simulink subsystem "Battery"  (R2025a)
settings: Solver=VariableStepAuto  StartTime=0.0  StopTime=10  RelTol=1e-3
model mask{minSOC=0, maxSOC=0, energyRating=0, capacityRating=0, nominalVoltage=0, frequency=0, windingRatio=0}
  mask prompts: minSOC "Minimum Operating SOC"; maxSOC "Maximum Operating SOC"; energyRating "Energy rating (kWh)"; capacityRating "Capacity Rating (Ah)"; nominalVoltage "Nominal Voltage (V)"; frequency "Frequency (Hz)"; windingRatio "Transformer Ratio"
libraries: fl_lib x13, ee_lib x6, nesl_utility x5, simulink x2, batteryecm_lib x1, eeGeneralControl x1
settings Model: DefaultTestHarness=Battery_Harness  Creator=skota  LastModifiedBy=skota

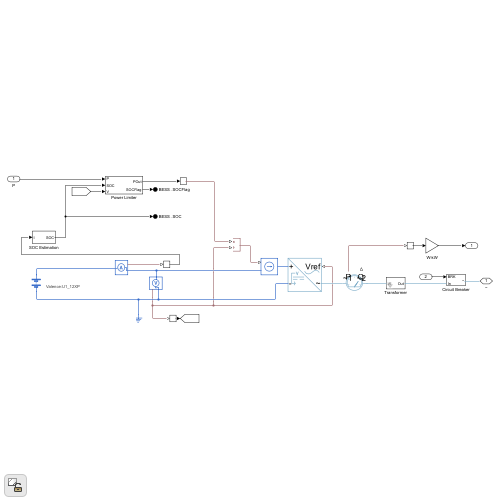
[thumbnail: Simulink's stored preview of the top-level diagram]
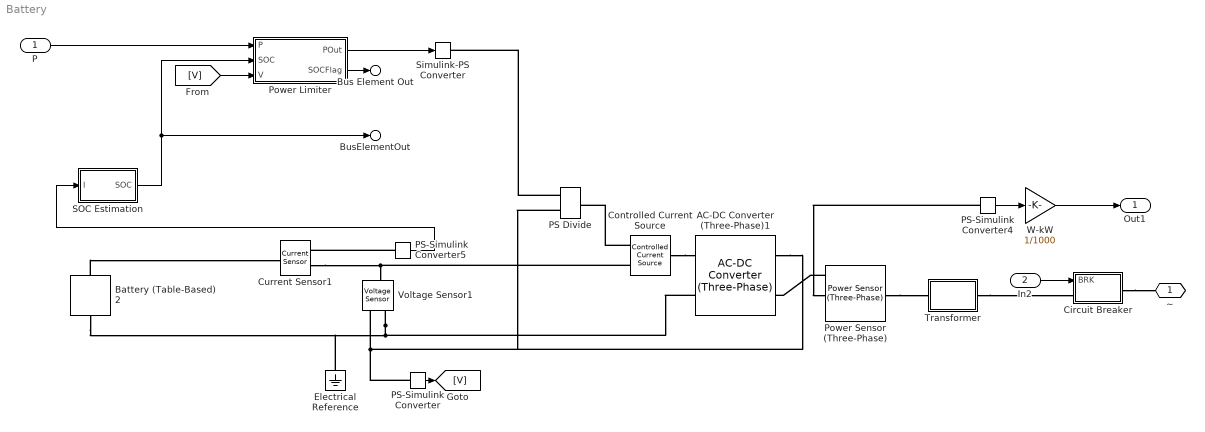
== system Battery ==
  P : Inport
  In2 : Inport  Port=2
  AC-DC Converter (Three-Phase)1 : ee_lib/Semiconductors & Converters/Converters/AC-DC Converter (Three-Phase)  port_option=ee.enum.threePhasePort.composite  droop=0.001 V/A  Vdc_dynamics=ee.enum.converters.dynamics.no  tauVdc=0.02 s  Vdc_ini=100 V  FRated=frequency Hz  Vline_rms_min=0.1 V  tauVac=1e-3 s  Vline_rms_ini=10000 V  Vang_ini=0 deg  power_dynamics=ee.enum.converters.powerDynamics.no  tauP=0.01 s  P_ini=1e3 W  gmin=1e-4 S
      settings: InternalSimscapePortConfiguration="{\"Bottom\":[],\"Left\":[{\"id\":\"Vref\",\"label\":\"Vref\",\"type\":\"input\"},{\"id\":\"N\",\"label\":\"~\",\"type\":\"foundation.electrical.three_phase\"}],\"Right\":[{\"id\":\"p\",\"label\":\"+\",\"type\":\"foundation.electrical.electrical\"},{\"id\":\"n\",\"label\":\"-\",\"type\":\"foundation.electrical.electrical\"}],\"Top\":[]}"
  Battery (Table-Based)2 : batteryecm_lib/Battery (Table-Based)  Tag={'toolbox/physmod/battery/shared_library/m/batteryecm_lib_parts';'Battery__Table_Based_/Valence/U1_12XP.xml'}  SOC_vec=[0 0.01 0.02 0.03 0.04 0.05 0.06 0.07 0.08 0.09 0.1 0.11 0.12 0.13 0.14 0.15 0.16 0.17 0.18 0.19 0.2 0.21 0.22 0.23 0.24 0.25 0.26 0.27 0.28 0.29 0.3 0.31 0.32 0.33 0.34 0.35 0.36 0.37 0.38 0.39 0.4 0.41 0.42 0.43 0.44 0.45 0.46 0.47 0.48 0.49 0.5 0.51 0.52 0.53 0.54 0.55 0.56 0.57 0.58 0.59 0.6 0.61 0.62 0.63 0.64 0.65 0.66 0.67 0.68 0.69 0.7 0.71 0.72 0.73 0.74 0.75 0.76 0.77 0.78 0.79 0.8 0.81 0.82 0.83 0.84 0.85 0.86 0.87 0.88 0.89 0.9 0.91 0.92 0.93 0.94 0.95 0.96 0.97 0.98 0.99 1]  T_dependence=simscape.enum.tablebattery.temperature_dependence.no  prm_dir=simscape.enum.tablebattery.prm_dir.noCurrentDirectionality  T_vec=[-10 0 10 20 23 30 40] degC  V0_mat=[12.00518 12.00518 12.00518 12.00518 12.00518 12.00518 12.00518;12.046 12.046 12.046 12.046 12.046 12.046 12.046;12.08682 12.08682 12.08682 12.08682 12.08682 12.08682 12.08682;12.12763 12.12763 12.12763 12.12763 12.12763 12.12763 12.12763;12.16845 12.16845 12.16845 12.16845 12.16845 12.16845 12.16845;12.20927 12.20927 12.20927 12.20927 12.20927 12.20927 12.20927;12.25009 12.25009 12.25009 12.25009 12.25009 12.25009 12.25009;12.29091 12.29091 12.29091 12.29091 12.29091 12.29091 12.29091;12.33173 12.33173 12.33173 12.33173 12.33173 12.33173 12.33173;12.37255 12.37255 12.37255 12.37255 12.37255 12.37255 12.37255;12.41337 12.41337 12.41337 12.41337 12.41337 12.41337 12.41337;12.45419 12.45419 12.45419 12.45419 12.45419 12.45419 12.45419;12.49501 12.49501 12.49501 12.49501 12.49501 12.49501 12.49501;12.53583 12.53583 12.53583 12.53583 12.53583 12.53583 12.53583;12.56952 12.56952 12.56952 12.56952 12.56952 12.56952 12.56952;12.60149 12.60149 12.60149 12.60149 12.60149 12.60149 12.60149;12.63628 12.63628 12.63628 12.63628 12.63628 12.63628 12.63628;12.66676 12.66676 12.66676 12.66676 12.66676 12.66676 12.66676;12.6925 12.6925 12.6925 12.6925 12.6925 12.6925 12.6925;12.71984 12.71984 12.71984 12.71984 12.71984 12.71984 12.71984;12.74668 12.74668 12.74668 12.74668 12.74668 12.74668 12.74668;12.7709 12.7709 12.7709 12.7709 12.7709 12.7709 12.7709;12.79145 12.79145 12.79145 12.79145 12.79145 12.79145 12.79145;12.81167 12.81167 12.81167 12.81167 12.81167 12.81167 12.81167;12.82987 12.82987 12.82987 12.82987 12.82987 12.82987 12.82987;12.84554 12.84554 12.84554 12.84554 12.84554 12.84554 12.84554;12.85927 12.85927 12.85927 12.85927 12.85927 12.85927 12.85927;12.87336 12.87336 12.87336 12.87336 12.87336 12.87336 12.87336;12.8878 12.8878 12.8878 12.8878 12.8878 12.8878 12.8878;12.90226 12.90226 12.90226 12.90226 12.90226 12.90226 12.90226;12.91618 12.91618 12.91618 12.91618 12.91618 12.91618 12.91618;12.92892 12.92892 12.92892 12.92892 12.92892 12.92892 12.92892;12.9409 12.9409 12.9409 12.9409 12.9409 12.9409 12.9409;12.95179 12.95179 12.95179 12.95179 12.95179 12.95179 12.95179;12.96212 12.96212 12.96212 12.96212 12.96212 12.96212 12.96212;12.9718 12.9718 12.9718 12.9718 12.9718 12.9718 12.9718;12.98121 12.98121 12.98121 12.98121 12.98121 12.98121 12.98121;12.9894 12.9894 12.9894 12.9894 12.9894 12.9894 12.9894;12.99628 12.99628 12.99628 12.99628 12.99628 12.99628 12.99628;13.00194 13.00194 13.00194 13.00194 13.00194 13.00194 13.00194;13.00687 13.00687 13.00687 13.00687 13.00687 13.00687 13.00687;13.01127 13.01127 13.01127 13.01127 13.01127 13.01127 13.01127;13.01612 13.01612 13.01612 13.01612 13.01612 13.01612 13.01612;13.0201 13.0201 13.0201 13.0201 13.0201 13.0201 13.0201;13.0231 13.0231 13.0231 13.0231 13.0231 13.0231 13.0231;13.0261 13.0261 13.0261 13.0261 13.0261 13.0261 13.0261;13.02911 13.02911 13.02911 13.02911 13.02911 13.02911 13.02911;13.03211 13.03211 13.03211 13.03211 13.03211 13.03211 13.03211;13.03451 13.03451 13.03451 13.03451 13.03451 13.03451 13.03451;13.03664 13.03664 13.03664 13.03664 13.03664 13.03664 13.03664;13.03933 13.03933 13.03933 13.03933 13.03933 13.03933 13.03933;13.04232 13.04232 13.04232 13.04232 13.04232 13.04232 13.04232;13.04573 13.04573 13.04573 13.04573 13.04573 13.04573 13.04573;13.04919 13.04919 13.04919 13.04919 13.04919 13.04919 13.04919;13.05277 13.05277 13.05277 13.05277 13.05277 13.05277 13.05277;13.05642 13.05642 13.05642 13.05642 13.05642 13.05642 13.05642;13.06013 13.06013 13.06013 13.06013 13.06013 13.06013 13.06013;13.06395 13.06395 13.06395 13.06395 13.06395 13.06395 13.06395;13.06828 13.06828 13.06828 13.06828 13.06828 13.06828 13.06828;13.07261 13.07261 13.07261 13.07261 13.07261 13.07261 13.07261;13.07686 13.07686 13.07686 13.07686 13.07686 13.07686 13.07686;13.08121 13.08121 13.08121 13.08121 13.08121 13.08121 13.08121;13.08594 13.08594 13.08594 13.08594 13.08594 13.08594 13.08594;13.09142 13.09142 13.09142 13.09142 13.09142 13.09142 13.09142;13.09708 13.09708 13.09708 13.09708 ...(+2253 chars)] V  V0_vec=[12.00518 12.046 12.08682 12.12763 12.16845 12.20927 12.25009 12.29091 12.33173 12.37255 12.41337 12.45419 12.49501 12.53583 12.56952 12.60149 12.63628 12.66676 12.6925 12.71984 12.74668 12.7709 12.79145 12.81167 12.82987 12.84554 12.85927 12.87336 12.8878 12.90226 12.91618 12.92892 12.9409 12.95179 12.96212 12.9718 12.98121 12.9894 12.99628 13.00194 13.00687 13.01127 13.01612 13.0201 13.0231 13.0261 13.02911 13.03211 13.03451 13.03664 13.03933 13.04232 13.04573 13.04919 13.05277 13.05642 13.06013 13.06395 13.06828 13.07261 13.07686 13.08121 13.08594 13.09142 13.09708 13.10279 13.10857 13.11438 13.12019 13.1263 13.13263 13.13899 13.14595 13.15268 13.15967 13.16669 13.17384 13.17943 13.18402 13.18838 13.19255 13.19694 13.20123 13.20527 13.20912 13.2115 13.21389 13.21588 13.21758 13.21949 13.22126 13.224 13.227 13.23066 13.23444 13.23732 13.23875 13.23911 13.23888 13.25149 13.31471]*100 V  V_range=[9 Inf] V  R0_mat=[0.31149 0.24646 0.1305 0.14557 0.06981 0.12094 0.10043;0.31245 0.23652 0.11852 0.12502 0.0625 0.09416 0.06761;0.30299 0.22658 0.10654 0.10446 0.05518 0.071 0.05004;0.29352 0.21664 0.09456 0.08497 0.04785 0.05545 0.03565;0.28405 0.2067 0.08326 0.0695 0.04083 0.04376 0.02394;0.27458 0.19676 0.07425 0.05748 0.03437 0.03259 0.01541;0.26512 0.18683 0.06508 0.0482 0.02911 0.02462 0.00923;0.25565 0.17689 0.05699 0.04095 0.02515 0.01945 0.00517;0.24618 0.16695 0.05025 0.03428 0.02195 0.01534 0.00236;0.23671 0.15701 0.04492 0.02949 0.01956 0.0115 0.00085;0.22724 0.14707 0.04118 0.02542 0.01764 0.00986 0.00061;0.21778 0.13713 0.03744 0.02233 0.01618 0.00823 0.00064;0.20831 0.12719 0.03369 0.01978 0.01518 0.00787 0.00119;0.19884 0.11725 0.03108 0.01847 0.01436 0.00758 0.00174;0.18937 0.10701 0.0287 0.01681 0.01349 0.00698 0.00186;0.1799 0.09743 0.02624 0.01521 0.01311 0.00656 0.00189;0.17044 0.08843 0.02418 0.01493 0.01277 0.00629 0.00207;0.16097 0.08111 0.0236 0.01443 0.01245 0.00644 0.00225;0.1515 0.074 0.02279 0.01369 0.01206 0.00666 0.00245;0.14203 0.0677 0.02206 0.01303 0.01189 0.00696 0.00273;0.13257 0.06168 0.0213 0.01283 0.01179 0.00725 0.00299;0.12217 0.05582 0.02087 0.01288 0.01168 0.00749 0.00323;0.11213 0.0525 0.02085 0.01275 0.01153 0.00754 0.00344;0.10314 0.04948 0.02082 0.0126 0.01152 0.00757 0.00364;0.09444 0.04636 0.02069 0.01235 0.01151 0.0075 0.00376;0.08561 0.04418 0.02043 0.01214 0.01146 0.00748 0.0039;0.07908 0.04215 0.02007 0.01218 0.0114 0.00741 0.00395;0.073 0.04014 0.01973 0.01225 0.01137 0.00737 0.00401;0.06878 0.03834 0.01964 0.01233 0.01137 0.00734 0.00403;0.06496 0.03708 0.01958 0.01241 0.01138 0.00731 0.00405;0.06117 0.0358 0.01949 0.01246 0.0114 0.00726 0.00405;0.05837 0.03446 0.01935 0.01262 0.01143 0.00716 0.00415;0.05554 0.0331 0.01917 0.01274 0.01146 0.00743 0.00426;0.05334 0.0326 0.01893 0.01281 0.01148 0.00765 0.00437;0.05171 0.03208 0.01888 0.01285 0.01149 0.00784 0.00451;0.05005 0.03152 0.01897 0.01286 0.0115 0.00799 0.00462;0.04837 0.03123 0.01906 0.01285 0.01151 0.00813 0.00474;0.04707 0.03089 0.01908 0.01288 0.01153 0.00821 0.00481;0.04632 0.03049 0.01903 0.01286 0.01152 0.00823 0.00482;0.04552 0.03007 0.01892 0.01278 0.0115 0.00818 0.00477;0.04468 0.02982 0.01878 0.01267 0.01147 0.00814 0.00471;0.04381 0.02954 0.01861 0.01253 0.01143 0.00809 0.00463;0.04296 0.02929 0.01847 0.01241 0.01141 0.00807 0.00457;0.04221 0.02899 0.0184 0.01224 0.01138 0.008 0.00447;0.04182 0.02866 0.01828 0.01203 0.01134 0.00789 0.00432;0.04143 0.02837 0.01816 0.01182 0.0113 0.00777 0.00417;0.04103 0.02807 0.01804 0.01172 0.01126 0.00767 0.00402;0.04064 0.02778 0.01792 0.01163 0.01122 0.00757 0.00401;0.04022 0.02746 0.01777 0.0115 0.01117 0.00745 0.00397;0.03979 0.02712 0.0176 0.01136 0.01113 0.00731 0.00391;0.03964 0.02688 0.01747 0.01125 0.0111 0.0072 0.00389;0.03949 0.02672 0.01735 0.01116 0.01108 0.0071 0.00387;0.03937 0.02658 0.01725 0.01108 0.01106 0.00705 0.00387;0.03925 0.02644 0.01717 0.01101 0.01105 0.00699 0.00387;0.03914 0.02631 0.01711 0.01094 0.01104 0.00695 0.00385;0.03903 0.02618 0.01705 0.01092 0.01103 0.0069 0.00384;0.03892 0.0262 0.017 0.01089 0.01102 0.00686 0.00382;0.03882 0.02624 0.01695 0.01087 0.01101 0.00683 0.00382;0.03877 0.02629 0.01693 0.01088 0.01102 0.00683 0.00387;0.0389 0.02635 0.01691 0.01089 0.01104 0.00684 0.00391;0.03901 0.0264 0.01689 0.01089 0.01105 0.00685 0.00396;0.03914 0.02644 0.01687 0.0109 0.01107 0.00686 0.004;0.03928 0.02648 0.01687 0.01093 0.01109 0.00689 0.00407;0.03946 0.02656 0.01694 0.011 0.01113 0.00695 0.00415;0.03965 0.02665 0.01709 0.01108 0.01117 0.00703 0.00425;0.03995 0.02674 0.01724 0.01117 0.01122 0.00714 0.00434;0.04035 0.02683 0.01739 0.01126 0.01127 0.00725 0.00443;0.04075 0.02692 0.01754 0.01136 0.01131 0.00736 0.00452;0.04115 0.02711 0.0177 0.01145 0.01136 0.00747 0.00461;0.04157 0.02734 0.01787 0.01156 0.01142 0.00759 0.00472;0.04196 0.02759 0.01803 0.01168 0.01148 0.00773 0.00483;0.04232 0.02783 0.01813 0.01181 0.01153 0.00786 0.00495;0.04271 0.02811 ...(+1584 chars)] Ohm  R0_vec=[0.06981 0.0625 0.05518 0.04785 0.04083 0.03437 0.02911 0.02515 0.02195 0.01956 0.01764 0.01618 0.01518 0.01436 0.01349 0.01311 0.01277 0.01245 0.01206 0.01189 0.01179 0.01168 0.01153 0.01152 0.01151 0.01146 0.0114 0.01137 0.01137 0.01138 0.0114 0.01143 0.01146 0.01148 0.01149 0.0115 0.01151 0.01153 0.01152 0.0115 0.01147 0.01143 0.01141 0.01138 0.01134 0.0113 0.01126 0.01122 0.01117 0.01113 0.0111 0.01108 0.01106 0.01105 0.01104 0.01103 0.01102 0.01101 0.01102 0.01104 0.01105 0.01107 0.01109 0.01113 0.01117 0.01122 0.01127 0.01131 0.01136 0.01142 0.01148 0.01153 0.0116 0.01166 0.01174 0.01182 0.0119 0.01195 0.012 0.01204 0.01209 0.01214 0.01219 0.01223 0.01227 0.01226 0.01225 0.01223 0.01221 0.01217 0.01212 0.01208 0.01205 0.01201 0.01196 0.01184 0.0117 0.01136 0.01069 0.0098 0.00774] Ohm  R0_dis_mat=[.0117, .0085, .009; .011, .0085, .009; .0114, .0087, .0092; .0107, .0082, .0088; .0107, .0083, .0091; .0113, .0085, .0089; .0116, .0085, .0089] % Parameter not set Ohm  R0_dis_vec=[.0085, .0085, .0087, .0082, .0083, .0085, .0085] % Parameter not set Ohm  R0_ch_mat=[.0117, .0085, .009; .011, .0085, .009; .0114, .0087, .0092; .0107, .0082, .0088; .0107, .0083, .0091; .0113, .0085, .0089; .0116, .0085, .0089] % Parameter not set Ohm  R0_ch_vec=[.0085, .0085, .0087, .0082, .0083, .0085, .0085] % Parameter not set Ohm  AH=40.779*ceil(energyRating*1000/(nominalVoltage*capacityRating)) hr*A  prm_leak=simscape.enum.tablebattery.prm_leak.disabled  Rleak_vec=[8000, 7000, 6000] % Parameter not set Ohm  Rleak=7e3 % Parameter not set Ohm  extrapolation_option=simscape.enum.extrapolation.nearest  SOC_port=simscape.enum.tablebattery.enable.no  prm_dyn=simscape.enum.tablebattery.prm_dyn.off  R1_mat=[.0109, .0029, .0013; .0069, .0024, .0012; .0047, .0026, .0013; .0034, .0016, .001; .0033, .0023, .0014; .0033, .0018, .0011; .0028, .0017, .0011] % Parameter not set Ohm  R1_vec=[.0029, .0024, .0026, .0016, .0023, .0018, .0017] % Parameter not set Ohm  tau1_mat=[20, 36, 39; 31, 45, 39; 109, 105, 61; 36, 29, 26; 59, 77, 67; 40, 33, 29; 25, 39, 33] % Parameter not set s  tau1_vec=[36, 45, 105, 29, 77, 33, 39] % Parameter not set s  R2_mat=[.0109, .0029, .0013; .0069, .0024, .0012; .0047, .0026, .0013; .0034, .0016, .001; .0033, .0023, .0014; .0033, .0018, .0011; .0028, .0017, .0011] % Parameter not set Ohm  R2_vec=[.0029, .0024, .0026, .0016, .0023, .0018, .0017] % Parameter not set Ohm  tau2_mat=[20, 36, 39; 31, 45, 39; 109, 105, 61; 36, 29, 26; 59, 77, 67; 40, 33, 29; 25, 39, 33] % Parameter not set s  tau2_vec=[36, 45, 105, 29, 77, 33, 39] % Parameter not set s  R3_mat=[.0109, .0029, .0013; .0069, .0024, .0012; .0047, .0026, .0013; .0034, .0016, .001; .0033, .0023, .0014; .0033, .0018, .0011; .0028, .0017, .0011] % Parameter not set Ohm  R3_vec=[.0029, .0024, .0026, .0016, .0023, .0018, .0017] % Parameter not set Ohm  tau3_mat=[20, 36, 39; 31, 45, 39; 109, 105, 61; 36, 29, 26; 59, 77, 67; 40, 33, 29; 25, 39, 33] % Parameter not set s  tau3_vec=[36, 45, 105, 29, 77, 33, 39] % Parameter not set s  R4_mat=[.0109, .0029, .0013; .0069, .0024, .0012; .0047, .0026, .0013; .0034, .0016, .001; .0033, .0023, .0014; .0033, .0018, .0011; .0028, .0017, .0011] % Parameter not set Ohm  R4_vec=[.0029, .0024, .0026, .0016, .0023, .0018, .0017] % Parameter not set Ohm  tau4_mat=[20, 36, 39; 31, 45, 39; 109, 105, 61; 36, 29, 26; 59, 77, 67; 40, 33, 29; 25, 39, 33] % Parameter not set s  tau4_vec=[36, 45, 105, 29, 77, 33, 39] % Parameter not set s  R5_mat=[.0109, .0029, .0013; .0069, .0024, .0012; .0047, .0026, .0013; .0034, .0016, .001; .0033, .0023, .0014; .0033, .0018, .0011; .0028, .0017, .0011] % Parameter not set Ohm  R5_vec=[.0029, .0024, .0026, .0016, .0023, .0018, .0017] % Parameter not set Ohm  tau5_mat=[20, 36, 39; 31, 45, 39; 109, 105, 61; 36, 29, 26; 59, 77, 67; 40, 33, 29; 25, 39, 33] % Parameter not set s  tau5_vec=[36, 45, 105, 29, 77, 33, 39] % Parameter not set s  prm_fade=simscape.enum.tablebattery.prm_fade.disabled  N0=100 % Parameter not set  dV0=0 % Parameter not set  dR0=0 % Parameter not set  dAH=0 % Parameter not set  dRleak=0 % Parameter not set  dR1=0 % Parameter not set  dR2=0 % Parameter not set  dR3=0 % Parameter not set  dR4=0 % Parameter not set  dR5=0 % Parameter not set  N0vec=[0 49 97 145 193 241 289 337 385 433 481 529 577 625 673 721 769 817 865 913 961 1009 1057 1105 1153 1201 1249 1297 1345 1393 1441 1489 1537 1585 1633 1681 1729 1777 1825 1873 1921 1969 2017 2065 2113 2161 2209 2257 2305 2353 2401 2449 2497 2545 2593 2641 2689 2737 2785 2833 2881 2929 2977 3025 3073 3121 3169 3217 3265 3313 3361 3409 3457 3505 3553 3601 3649 3697 3745 3793 3841 3889 3937 3985 4033 4081 4129 4177 4225 4273 4321 4369 4417 4465 4513 4561 4609 4657 4705 4753]  Tfadevec=[298.15, 323.15] % Parameter not set K  dV0vec=[0 -0.2242 -0.4483 -0.5142 -0.5589 -0.569 -0.5683 -0.5681 -0.5692 -0.5703 -0.5741 -0.5782 -0.5834 -0.5917 -0.6 -0.6099 -0.6207 -0.6305 -0.6399 -0.6492 -0.6586 -0.6663 -0.6741 -0.6817 -0.6907 -0.7003 -0.707 -0.7132 -0.7197 -0.7264 -0.7327 -0.7387 -0.7438 -0.7496 -0.7554 -0.7619 -0.7688 -0.7757 -0.7826 -0.7901 -0.8006 -0.813 -0.8255 -0.8384 -0.8519 -0.8664 -0.881 -0.8958 -0.9106 -0.9251 -0.9392 -0.9546 -0.972 -0.9899 -1.0083 -1.029 -1.0514 -1.0782 -1.1068 -1.135 -1.1599 -1.1836 -1.2073 -1.2304 -1.2531 -1.2762 -1.2997 -1.323 -1.3445 -1.366 -1.3874 -1.4088 -1.4297 -1.4544 -1.4788 -1.5029 -1.5269 -1.5509 -1.5749 -1.5987 -1.6223 -1.6459 -1.6686 -1.6899 -1.711 -1.7302 -1.7484 -1.7656 -1.7823 -1.7987 -1.8151 -1.8379 -1.8631 -1.8878 -1.9102 -1.9319 -1.9533 -1.9745 -1.9953 -2.0155]  dR0vec=[0 0 0 0 0 0 0 0 0 0 0 0 0 0 0 0 0 0 0 0 0 0 0 0 0 0 0 0 0 0 0 0 0 0 0 0 0 0 0 0 0 0 0 0 0 0 0 0 0 0 0 0 0 0 0 0 0 0 0 0 0 0 0 0 0 0 0 0 0 0 0 0 0 0 0 0 0 0 0 0 0 0 0 0 0 0 0 0 0 0 0 0 0 0 0 0 0 0 0 0] % Parameter assumed  dAHvec=[0 -0.472 -0.944 -1.416 -1.889 -2.306 -2.716 -3.125 -3.535 -3.944 -4.342 -4.723 -5.104 -5.485 -5.867 -6.248 -6.629 -6.972 -7.314 -7.656 -7.997 -8.339 -8.681 -9.022 -9.457 -9.923 -10.389 -10.855 -11.321 -11.787 -12.254 -12.72 -13.106 -13.491 -13.876 -14.262 -14.647 -15.032 -15.417 -15.837 -16.264 -16.69 -17.116 -17.542 -17.987 -18.438 -18.889 -19.341 -19.792 -20.243 -20.694 -21.177 -21.71 -22.243 -22.776 -23.309 -23.842 -24.376 -24.909 -25.442 -25.915 -26.366 -26.816 -27.266 -27.717 -28.167 -28.617 -29.068 -29.518 -29.968 -30.419 -30.869 -31.319 -31.858 -32.41 -32.961 -33.512 -34.063 -34.615 -35.166 -35.717 -36.269 -36.802 -37.314 -37.826 -38.339 -38.851 -39.363 -39.875 -40.388 -40.9 -41.603 -42.38 -43.158 -43.935 -44.712 -45.49 -46.267 -47.044 -47.822]  dRleakvec=[0, 0, 0, 0] % Parameter not set  dR1vec=[0, 0, 0, 0] % Parameter not set  dR2vec=[0, 0, 0, 0] % Parameter not set  dR3vec=[0, 0, 0, 0] % Parameter not set  dR4vec=[0, 0, 0, 0] % Parameter not set  dR5vec=[0, 0, 0, 0] % Parameter not set  dV0mat=[0, 0; 0, 0; 0, 0; 0, 0] % Parameter not set  dR0mat=[0, 0; 0, 0; 0, 0; 0, 0] % Parameter not set  dAHmat=[0, 0; 0, 0; 0, 0; 0, 0] % Parameter not set  dRleakmat=[0, 0; 0, 0; 0, 0; 0, 0] % Parameter not set  dR1mat=[0, 0; 0, 0; 0, 0; 0, 0] % Parameter not set  dR2mat=[0, 0; 0, 0; 0, 0; 0, 0] % Parameter not set  dR3mat=[0, 0; 0, 0; 0, 0; 0, 0] % Parameter not set  dR4mat=[0, 0; 0, 0; 0, 0; 0, 0] % Parameter not set  dR5mat=[0, 0; 0, 0; 0, 0; 0, 0] % Parameter not set  prm_age_modeling=simscape.enum.tablebattery.prm_age_modeling.equation  storage_dt_age_vec=[0] % Parameter not set d  storage_T_age_vec=[273] % Parameter not set K  prm_age_OCV=simscape.enum.tablebattery.prm_age_OCV.OCV  OCV_age=0.9 % Parameter not set  SOC_age=0.6 % Parameter not set  prm_age_resistance=simscape.enum.tablebattery.prm_age.disabled  OCV_scaling_age_resistance=2.2134e6 % Parameter not set  OCV_offset_age_resistance=1.632e6 % Parameter not set  temp_exp_age_resistance=0.515833569 % Parameter not set V  t_exp_age_resistance=0.75 % Parameter not set  T_age_vec_resistance=[273.15, 298.15, 323.15] % Parameter not set K  dt_age_vec_resistance=[0, 90, 180, 270] % Parameter not set d  dR0_age_vec=[0, 0, 0] % Parameter not set  t_meas_dR0_age=100 % Parameter not set d  dR0_age_mat=[0, 0, 0; 0, 0, 0; 0, 0, 0; 0, 0, 0] % Parameter not set  prm_age_capacity=simscape.enum.tablebattery.prm_age.disabled  OCV_scaling_age_capacity=1.5097e07 % Parameter not set  OCV_offset_age_capacity=8.3625e06 % Parameter not set  temp_exp_age_capacity=0.6011 % Parameter not set V  t_exp_age_capacity=0.75 % Parameter not set  T_age_vec_capacity=[273.15, 298.15, 323.15] % Parameter not set K  dt_age_vec_capacity=[0, 90, 180, 270] % Parameter not set d  dAH_age_vec=[0, 0, 0] % Parameter not set  t_meas_dAH_age=100 % Parameter not set d  dAH_age_mat=[0, 0, 0; 0, 0, 0; 0, 0, 0; 0, 0, 0] % Parameter not set  thermal_port=simscape.enum.thermaleffects.omit  temperature=298.15 % Parameter not set K  thermal_mass=5868 % Parameter assumed J/K  i_specify=off  i_priority=None  i=0 A  i_nominal_specify=off  i_nominal_value=1  i_nominal_unit=A  v_specify=off  v_priority=None  v=0 V  v_nominal_specify=off  v_nominal_value=1  v_nominal_unit=V  stateOfCharge_specify=on  stateOfCharge_priority=High  stateOfCharge=0.95  stateOfCharge_nominal_specify=off  stateOfCharge_nominal_value=1  stateOfCharge_nominal_unit=1  num_cycles_specify=off  num_cycles_priority=High  num_cycles=0  num_cycles_nominal_specify=off  num_cycles_nominal_value=1  num_cycles_nominal_unit=1  cell_temperature_specify=off  cell_temperature_priority=High  cell_temperature=298.15 K  cell_temperature_nominal_specify=off  cell_temperature_nominal_value=1  cell_temperature_nominal_unit=K
      settings: AttributesFormatString=Valence:U1_12XP  InternalSimscapePortConfiguration="{\"Bottom\":[],\"Left\":[{\"id\":\"p\",\"label\":\"+\",\"type\":\"foundation.electrical.electrical\"}],\"Right\":[{\"id\":\"n\",\"label\":\"-\",\"type\":\"foundation.electrical.electrical\"}],\"Top\":[]}"
  Circuit Breaker : Subsystem
  Controlled Current Source : fl_lib/Electrical/Electrical Sources/Controlled Current Source
  Current Sensor1 : fl_lib/Electrical/Electrical Sensors/Current Sensor
  Electrical Reference : fl_lib/Electrical/Electrical Elements/Electrical Reference
  PS Divide : fl_lib/Physical Signals/Functions/PS Divide
  PS-Simulink Converter : nesl_utility/PS-Simulink Converter  PhysicalDomain=network_engine_domain  SubClassName=ps_output  LeftPortType=input  RightPortType=output  PseudoPeriodic=off  Frequencies=[]  VectorFormat=inherit  Unit=inherit  AffineConversion=off
  PS-Simulink Converter4 : nesl_utility/PS-Simulink Converter  PhysicalDomain=network_engine_domain  SubClassName=ps_output  LeftPortType=input  RightPortType=output  PseudoPeriodic=off  Frequencies=[]  VectorFormat=inherit  Unit=inherit  AffineConversion=off
  PS-Simulink Converter5 : nesl_utility/PS-Simulink Converter  PhysicalDomain=network_engine_domain  SubClassName=ps_output  LeftPortType=input  RightPortType=output  PseudoPeriodic=off  Frequencies=[]  VectorFormat=inherit  Unit=inherit  AffineConversion=off
  Power Limiter : Subsystem
  Power Sensor (Three-Phase) : ee_lib/Sensors & Transducers/Power Sensor (Three-Phase)  load_type=ee.enum.passive.type_balanced.balanced  f0=60 Hz  config=ee.enum.with_neutral.no  rho=1
      settings: InternalSimscapePortConfiguration="{\"Bottom\":[],\"Left\":[{\"id\":\"N1\",\"label\":\"~1\",\"type\":\"foundation.electrical.three_phase\"}],\"Right\":[{\"id\":\"N2\",\"label\":\"~2\",\"type\":\"foundation.electrical.three_phase\"}],\"Top\":[{\"id\":\"Pm\",\"label\":\"P\",\"type\":\"output\"},{\"id\":\"Qm\",\"label\":\"Q\",\"type\":\"output\"}]}"
  SOC Estimation : Subsystem
  Simulink-PS Converter : nesl_utility/Simulink-PS Converter  PhysicalDomain=network_engine_domain  SubClassName=ps_input  LeftPortType=input  RightPortType=output  PseudoPeriodic=off  Frequencies=[]  NoiseDistribution=none  NoiseParameters=[]  Unit=V*A  AffineConversion=off  FilteringAndDerivatives=provide  SimscapeFilterOrder=1  InputFilterTimeConstant=0.001  UdotUserProvided=0
  Transformer : Subsystem  mask{windingRatio=windingRatio}
      mask prompts: windingRatio "Winding ratio"
      mask DialogControl Container4 Prompt: General
  Voltage Sensor1 : fl_lib/Electrical/Electrical Sensors/Voltage Sensor
  W-kW : Gain  Gain=1/1000
  ~ : PMIOPort  Side=Left
  Out1 : Outport
  Bus Element Out : Outport  Port=2  PortName=BESS  Element=SOCFlag
  BusElementOut : Outport  Port=2  PortName=BESS  Element=SOC
  wires:
  Power Limiter/1(POut) -> Simulink-PS Converter/1
  PS-Simulink Converter4/1 -> W-kW/1
  PS-Simulink Converter5/1 -> SOC Estimation/1(I)
  SOC Estimation/1(SOC) -> Power Limiter/2(SOC), BusElementOut/1
  In2/1 -> Circuit Breaker/1(BRK)
  Power Limiter/2(SOCFlag) -> Bus Element Out/1
  PS-Simulink Converter/1 -> [V]
  [V] -> Power Limiter/3(V)
  P/1 -> Power Limiter/1(P)
  W-kW/1 -> Out1/1
  connections:
  Controlled Current Source/RConn2 -- Voltage Sensor1/LConn1 -- Current Sensor1/RConn2
  PS-Simulink Converter/LConn1 -- AC-DC Converter (Three-Phase)1/LConn1 -- PS Divide/LConn2 -- Voltage Sensor1/RConn1
  Voltage Sensor1/RConn2 -- Battery (Table-Based)2/RConn1 -- Electrical Reference/LConn1 -- AC-DC Converter (Three-Phase)1/RConn2
  Power Sensor (Three-Phase)/LConn1 -- AC-DC Converter (Three-Phase)1/LConn2
  PS-Simulink Converter5/LConn1 -- Current Sensor1/RConn1
  Battery (Table-Based)2/LConn1 -- Current Sensor1/LConn1
  PS-Simulink Converter4/LConn1 -- Power Sensor (Three-Phase)/LConn2
  Controlled Current Source/LConn1 -- AC-DC Converter (Three-Phase)1/RConn1
  Controlled Current Source/RConn1 -- PS Divide/RConn1
  PS Divide/LConn1 -- Simulink-PS Converter/RConn1
  Circuit Breaker/RConn1 -- ~/RConn1
  Power Sensor (Three-Phase)/RConn1 -- Transformer/LConn1
  Transformer/RConn1 -- Circuit Breaker/LConn1

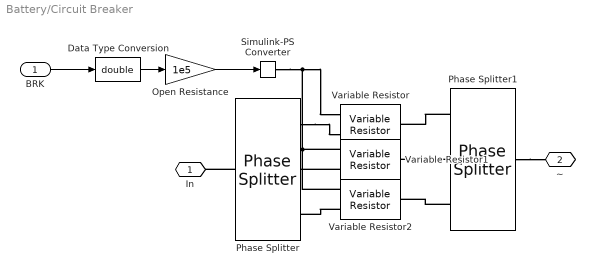
== system Battery/Circuit Breaker ==
  BRK : Inport
  Data Type Conversion : DataTypeConversion  OutDataTypeStr=double  SaturateOnIntegerOverflow=off  RndMeth=Floor
  Open Resistance : Gain  Gain=1e5
  Phase Splitter : ee_lib/Connectors & References/Phase Splitter
  Phase Splitter1 : ee_lib/Connectors & References/Phase Splitter
  Simulink-PS Converter : nesl_utility/Simulink-PS Converter  PhysicalDomain=network_engine_domain  SubClassName=ps_input  LeftPortType=input  RightPortType=output  PseudoPeriodic=off  Frequencies=[]  NoiseDistribution=none  NoiseParameters=[]  Unit=1  AffineConversion=off  FilteringAndDerivatives=provide  SimscapeFilterOrder=1  InputFilterTimeConstant=0.001  UdotUserProvided=0
  Variable Resistor : fl_lib/Electrical/Electrical Elements/Variable Resistor  Rmin=1e-4 Ohm  thermalEnable=false  thermal_mass=1 J/K  i_specify=off  i_priority=None  i=0 A  i_nominal_specify=off  i_nominal_value=1  i_nominal_unit=A  v_specify=off  v_priority=None  v=0 V  v_nominal_specify=off  v_nominal_value=1  v_nominal_unit=V  T_specify=off  T_priority=None  T=300 K  T_nominal_specify=off  T_nominal_value=1  T_nominal_unit=K
  Variable Resistor1 : fl_lib/Electrical/Electrical Elements/Variable Resistor  Rmin=1e-4 Ohm  thermalEnable=false  thermal_mass=1 J/K  i_specify=off  i_priority=None  i=0 A  i_nominal_specify=off  i_nominal_value=1  i_nominal_unit=A  v_specify=off  v_priority=None  v=0 V  v_nominal_specify=off  v_nominal_value=1  v_nominal_unit=V  T_specify=off  T_priority=None  T=300 K  T_nominal_specify=off  T_nominal_value=1  T_nominal_unit=K
  Variable Resistor2 : fl_lib/Electrical/Electrical Elements/Variable Resistor  Rmin=1e-4 Ohm  thermalEnable=false  thermal_mass=1 J/K  i_specify=off  i_priority=None  i=0 A  i_nominal_specify=off  i_nominal_value=1  i_nominal_unit=A  v_specify=off  v_priority=None  v=0 V  v_nominal_specify=off  v_nominal_value=1  v_nominal_unit=V  T_specify=off  T_priority=None  T=300 K  T_nominal_specify=off  T_nominal_value=1  T_nominal_unit=K
  In : PMIOPort  Side=Left
  ~ : PMIOPort  Port=2  Side=Right
  wires:
  Open Resistance/1 -> Simulink-PS Converter/1
  BRK/1 -> Data Type Conversion/1
  Data Type Conversion/1 -> Open Resistance/1
  connections:
  Phase Splitter/LConn1 -- In/RConn1
  Variable Resistor1/LConn1 -- Variable Resistor2/LConn1 -- Simulink-PS Converter/RConn1 -- Variable Resistor/LConn1
  Phase Splitter1/LConn1 -- ~/RConn1
  Phase Splitter1/RConn1 -- Variable Resistor/RConn1
  Variable Resistor2/LConn2 -- Phase Splitter/RConn3
  Phase Splitter/RConn1 -- Variable Resistor/LConn2
  Phase Splitter1/RConn3 -- Variable Resistor2/RConn1
  Variable Resistor1/LConn2 -- Phase Splitter/RConn2
  Phase Splitter1/RConn2 -- Variable Resistor1/RConn1

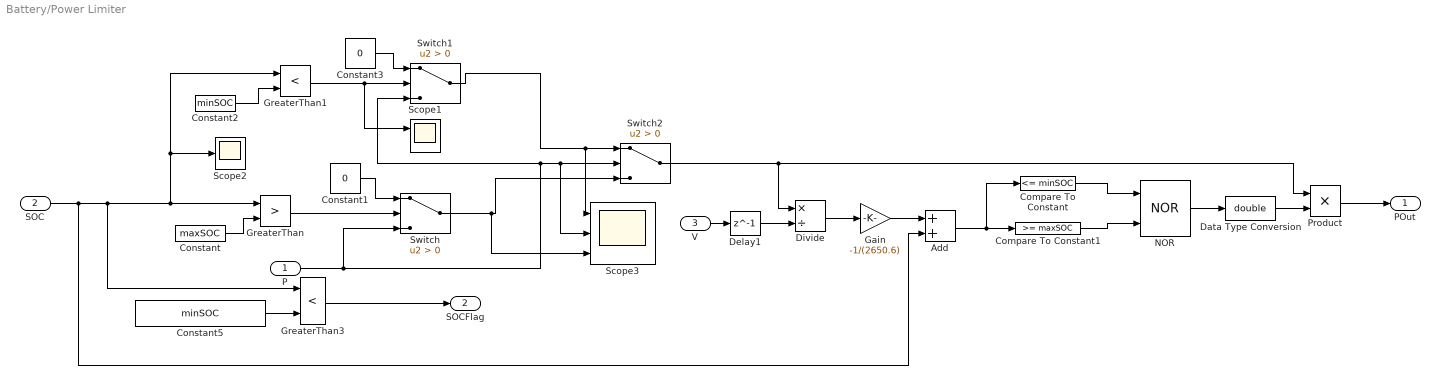
== system Battery/Power Limiter ==
  P : Inport
  SOC : Inport  Port=2
  V : Inport  Port=3
  Add : Sum
  Compare To Constant : simulink/Logic and Bit Operations/Compare To Constant  relop=<=  const=minSOC  OutDataTypeStr=boolean
  Compare To Constant1 : simulink/Logic and Bit Operations/Compare To Constant  relop=>=  const=maxSOC  OutDataTypeStr=boolean
  Constant : Constant  Value=maxSOC
  Constant1 : Constant  Value=0
  Constant2 : Constant  Value=minSOC
  Constant3 : Constant  Value=0
  Constant5 : Constant  Value=minSOC
  Data Type Conversion : DataTypeConversion  OutDataTypeStr=double  SaturateOnIntegerOverflow=off  RndMeth=Floor
  Delay1 : Delay  DelayLength=1
  Divide : Product  Inputs=*/
  Gain : Gain  Gain=-1/(2650.6)
  GreaterThan : RelationalOperator  Operator=>  OutDataTypeStr=boolean  RndMeth=Simplest  InputSameDT=off
  GreaterThan1 : RelationalOperator  Operator=<  OutDataTypeStr=boolean  RndMeth=Simplest  InputSameDT=off
  GreaterThan3 : RelationalOperator  Operator=<  OutDataTypeStr=boolean  RndMeth=Simplest  InputSameDT=off
  NOR : Logic  Operator=NOR  IconShape=distinctive  AllPortsSameDT=off  OutDataTypeStr=boolean
  Product : Product
  Scope1 : Scope  NumInputPorts=2
  Scope2 : Scope
  Scope3 : Scope  NumInputPorts=3
  Switch : Switch  Criteria=u2 > Threshold  SaturateOnIntegerOverflow=off  InputSameDT=off
  Switch1 : Switch  Criteria=u2 > Threshold  SaturateOnIntegerOverflow=off  InputSameDT=off
  Switch2 : Switch  Criteria=u2 > Threshold  SaturateOnIntegerOverflow=off  InputSameDT=off
  POut : Outport
  SOCFlag : Outport  Port=2
  wires:
  Product/1 -> POut/1
  Gain/1 -> Add/1
  Data Type Conversion/1 -> Product/2
  NOR/1 -> Data Type Conversion/1
  Compare To Constant1/1 -> NOR/2
  Compare To Constant/1 -> NOR/1
  Add/1 -> Compare To Constant1/1, Compare To Constant/1
  Switch2/1 -> Product/1, Divide/1
  Switch/1 -> Switch2/3, Scope3/3
  SOC/1 -> GreaterThan/1, GreaterThan1/1, Scope2/1, GreaterThan3/1, Add/2
  Divide/1 -> Gain/1
  Delay1/1 -> Divide/2
  V/1 -> Delay1/1
  GreaterThan3/1 -> SOCFlag/1
  Constant5/1 -> GreaterThan3/2
  Constant/1 -> GreaterThan/2
  GreaterThan/1 -> Switch/2
  Constant1/1 -> Switch/1
  Constant2/1 -> GreaterThan1/2
  GreaterThan1/1 -> Switch1/2, Scope1/1
  Constant3/1 -> Switch1/1
  Switch1/1 -> Switch2/1, Scope3/1
  P/1 -> Switch/3, Switch1/3, Switch2/2, Scope3/2

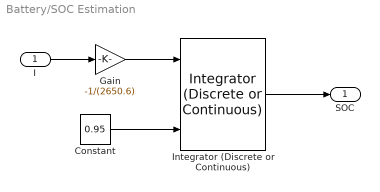
== system Battery/SOC Estimation ==
  I : Inport
  Constant : Constant  Value=0.95
  Gain : Gain  Gain=-1/(2650.6)
  Integrator (Discrete or Continuous) : eeGeneralControl/Integrator (Discrete or Continuous)  LabelModeActiveChoice=Discrete  ExternalReset=level  LimitType=Anti-windup  B=inf  A=-inf  Ts=-1
      settings: LibrarySourceBlock=|
      | ee_sl_lib/General Control/Integrator
      | (Discrete or Continuous)
  SOC : Outport
  wires:
  Integrator (Discrete or Continuous)/1 -> SOC/1
  Gain/1 -> Integrator (Discrete or Continuous)/1
  I/1 -> Gain/1
  Constant/1 -> Integrator (Discrete or Continuous)/3

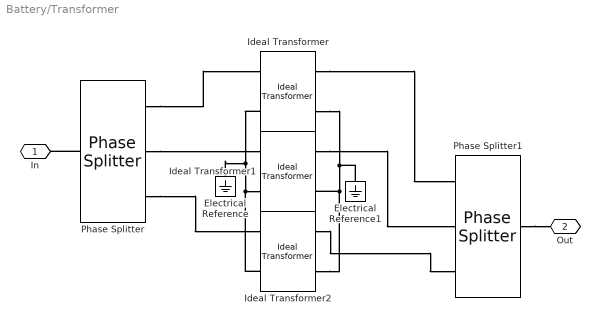
== system Battery/Transformer ==
  Electrical Reference : fl_lib/Electrical/Electrical Elements/Electrical Reference
  Electrical Reference1 : fl_lib/Electrical/Electrical Elements/Electrical Reference
  Ideal Transformer : fl_lib/Electrical/Electrical Elements/Ideal Transformer  n=windingRatio  i1_specify=off  i1_priority=None  i1=0 A  i1_nominal_specify=off  i1_nominal_value=1  i1_nominal_unit=A  v1_specify=off  v1_priority=None  v1=0 V  v1_nominal_specify=off  v1_nominal_value=1  v1_nominal_unit=V  i2_specify=off  i2_priority=None  i2=0 A  i2_nominal_specify=off  i2_nominal_value=1  i2_nominal_unit=A  v2_specify=off  v2_priority=None  v2=0 V  v2_nominal_specify=off  v2_nominal_value=1  v2_nominal_unit=V
  Ideal Transformer1 : fl_lib/Electrical/Electrical Elements/Ideal Transformer  n=windingRatio  i1_specify=off  i1_priority=None  i1=0 A  i1_nominal_specify=off  i1_nominal_value=1  i1_nominal_unit=A  v1_specify=off  v1_priority=None  v1=0 V  v1_nominal_specify=off  v1_nominal_value=1  v1_nominal_unit=V  i2_specify=off  i2_priority=None  i2=0 A  i2_nominal_specify=off  i2_nominal_value=1  i2_nominal_unit=A  v2_specify=off  v2_priority=None  v2=0 V  v2_nominal_specify=off  v2_nominal_value=1  v2_nominal_unit=V
  Ideal Transformer2 : fl_lib/Electrical/Electrical Elements/Ideal Transformer  n=windingRatio  i1_specify=off  i1_priority=None  i1=0 A  i1_nominal_specify=off  i1_nominal_value=1  i1_nominal_unit=A  v1_specify=off  v1_priority=None  v1=0 V  v1_nominal_specify=off  v1_nominal_value=1  v1_nominal_unit=V  i2_specify=off  i2_priority=None  i2=0 A  i2_nominal_specify=off  i2_nominal_value=1  i2_nominal_unit=A  v2_specify=off  v2_priority=None  v2=0 V  v2_nominal_specify=off  v2_nominal_value=1  v2_nominal_unit=V
  Phase Splitter : ee_lib/Connectors & References/Phase Splitter
  Phase Splitter1 : ee_lib/Connectors & References/Phase Splitter
  In : PMIOPort  Side=Left
  Out : PMIOPort  Port=2  Side=Right
  connections:
  Ideal Transformer/RConn2 -- Electrical Reference1/LConn1 -- Ideal Transformer1/RConn2 -- Ideal Transformer2/RConn2
  Phase Splitter/RConn3 -- Ideal Transformer2/LConn1
  Phase Splitter/RConn2 -- Ideal Transformer1/LConn1
  Phase Splitter/RConn1 -- Ideal Transformer/LConn1
  Ideal Transformer/LConn2 -- Electrical Reference/LConn1 -- Ideal Transformer1/LConn2 -- Ideal Transformer2/LConn2
  Phase Splitter/LConn1 -- In/RConn1
  Phase Splitter1/LConn1 -- Out/RConn1
  Ideal Transformer/RConn1 -- Phase Splitter1/RConn1
  Ideal Transformer2/RConn1 -- Phase Splitter1/RConn3
  Ideal Transformer1/RConn1 -- Phase Splitter1/RConn2
